simulink model "eye_animation"  (R2019a)
settings: Solver=FixedStepAuto  StartTime=0.0  StopTime=t_finish  FixedStep=fix_step_size  RelTol=1e-3
values from neighbouring files (symbols this model uses):
  fix_step_size = 0.001    [EyeScript.m]
  slow_time = 1    [EyeScript.m]    (also in animationscript.m)
undefined symbols (not defined in the file or in its folder): gray
libraries: vrlib x4
settings Model: Creator=murat  LastModifiedBy=murat

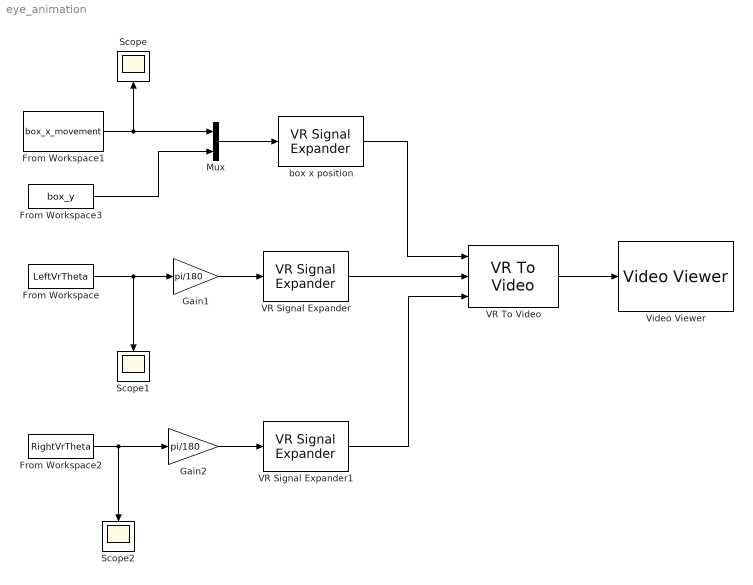
== system eye_animation ==
  From Workspace : FromWorkspace  VariableName=LeftVrTheta  SampleTime=0
  From Workspace1 : FromWorkspace  VariableName=box_x_movement  SampleTime=0
  From Workspace2 : FromWorkspace  VariableName=RightVrTheta  SampleTime=0
  From Workspace3 : FromWorkspace  VariableName=box_y  SampleTime=0
  Gain1 : Gain  Gain=pi/180
  Gain2 : Gain  Gain=pi/180
  Mux : Mux  Inputs=2
  Scope : Scope
  Scope1 : Scope
  Scope2 : Scope
  VR Signal Expander : vrlib/VR Signal Expander  outwidth=4  outidx=[4]
      settings: SourceProductName=Simulink
  VR Signal Expander1 : vrlib/VR Signal Expander  outwidth=4  outidx=[4]
      settings: SourceProductName=Simulink
  VR To Video : vrlib/VR To Video  InstantiateOnLoad=on  SampleTime=fix_step_size*50/slow_time  ViewEnable=on  RemoteChange=off  RemoteView=off  FieldsWritten=Box.translation.3.1.1.double#Eye_Left.rotation.4.1.1.double#Eye_Right.rotation.4.1.1.double  WorldFileName=eye3d.wrl  AutoView=off  VideoDimensions=[1080 1920]  AllowVariableSize=off
      settings: SourceProductName=Simulink  SourceProductBaseCode=SL
  Video Viewer : VideoViewer  colormapValue=gray(256)  FigPos=[1 822 1536 724]
  box x position : vrlib/VR Signal Expander  outwidth=3  outidx=[1 2]
      settings: SourceProductName=Simulink
  wires:
  From Workspace/1 -> Scope1/1, Gain1/1
  From Workspace1/1 -> Mux/1, Scope/1
  Gain1/1 -> VR Signal Expander/1
  Gain2/1 -> VR Signal Expander1/1
  From Workspace2/1 -> Scope2/1, Gain2/1
  Mux/1 -> box x position/1
  From Workspace3/1 -> Mux/2
  VR To Video/1 -> Video Viewer/1
  box x position/1 -> VR To Video/1
  VR Signal Expander/1 -> VR To Video/2
  VR Signal Expander1/1 -> VR To Video/3
